simulink model "RightArm"  (Simulink 6.5)
settings: Solver=ode45  SolverMode=SingleTasking  StartTime=0.0  StopTime=10.0  RelTol=1e-3  AbsTol=1e-6
settings Model: Creator=The MathWorks Inc.  LastModifiedBy=suarezjl  ExtModeTrigMode=oneshot  ExtModeArmWhenConnect=off  ExtModeAutoUpdateStatusClock=off
settings DataIOCC: LimitDataPoints=off  SignalLoggingName=logsOut
settings OptimizationCC: BooleanDataType=off  InlineInvariantSignals=on
settings DebuggingCC: CheckExecutionContextPreStartOutputMsg=on  CheckExecutionContextRuntimeOutputMsg=on  SolverPrmCheckMsg=none  MultiTaskDSMMsg=warning  MultiTaskCondExecSysMsg=none  IntegerOverflowMsg=none  StrictBusMsg=None
settings HardwareCC: TargetUnknown=on
settings ModelReferenceCC: UpdateModelReferenceTargets=IfOutOfDate
settings RTWCC: IncludeERTFirstTime=on

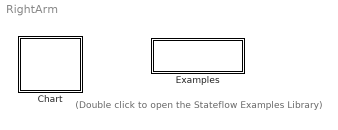
== system RightArm ==
  note: (Double click to open the
      | Stateflow Examples Library)
  Chart : Stateflow chart
  Examples : Subsystem
      settings: OpenFcn=sf('Private','sf_examples')
      mask Display: disp('Examples')

== system RightArm/Examples ==

== stateflow chart Chart ==
  state InitialArmRoutine
    Popeye\RightArm\HomingController.MoveThroughDexterousWorkspace()
    Popeye\RightArm\SampleIndPressure.HW_IO_12()
    Popeye\RightArm\StateMachine.Wait(200)
  state InitializeFunctions
    Popeye\RightArm\SampleIndPressure.Initialize()
    Popeye\RightArm\PIDNonLinCtrl.Initial()
    Popeye\RightArm\ForwardKinematics.Initialize()
    Popeye\RightArm\InverseKinematics.Initialize()
    Popeye\RightArm\SampleIndPressure.Disable_ZMasking()
  state Stop
    Popeye\RightArm\SampleIndPressure.Reset()
  (default) -> InitializeFunctions : Start
  InitialArmRoutine -> InitialArmRoutine [order 1] : Default
  InitializeFunctions -> InitialArmRoutine : Always
  InitialArmRoutine -> Stop [order 2] : Signal="Stop"
